simulink model "dual_heater"  (R2023b)
settings: Solver=VariableStepAuto  StartTime=0.0  StopTime=600  FixedStep=1  RelTol=1e-3
values from neighbouring files (symbols this model uses):
  A = 7e-4    (= 0.0007)    [dual_heater1.m]    (also in one_heater1.m = 0.0012)
  alfa = 0.01    [dual_heater1.m]    (also in one_heater1.m = 0.5)
  alfa2 = 0.0075    [dual_heater1.m]
  As = 5e-4    (= 0.0005)    [dual_heater1.m]
  C2K = 273.15    [dual_heater1.m]    (also in one_heater1.m)
  cp = 500    [dual_heater1.m]    (also in one_heater1.m)
  m = 4e-3    (= 0.004)    [dual_heater1.m]    (also in one_heater1.m)
  sig = 5.67e-8    (= 5.67e-08)    [dual_heater1.m]    (also in one_heater1.m)
  T = T + C2K    (= 296.15)    [dual_heater1.m]    (also in one_heater1.m)
  t0 = t0 + C2K    (= 296.15)    [dual_heater1.m]    (also in one_heater1.m)
  U = 10    [dual_heater1.m]    (also in one_heater1.m)
undefined symbols (not defined in the file or in its folder): pow
settings Model: Creator=ondre  LastModifiedBy=ondre

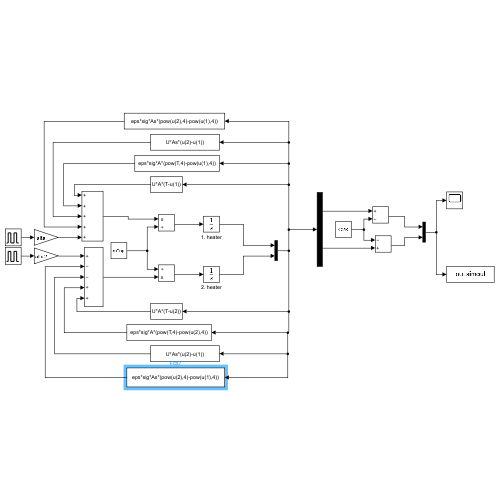
[thumbnail: Simulink's stored preview of the top-level diagram]
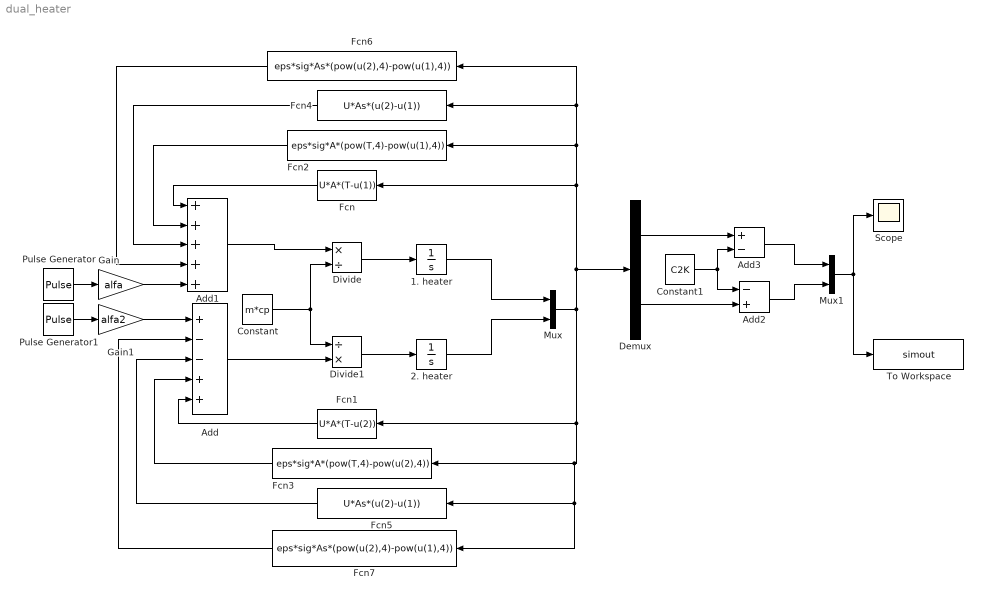
== system dual_heater ==
  1. heater : Integrator  InitialCondition=t0
  2. heater : Integrator  InitialCondition=t0
  Add : Sum  Inputs=+--++
  Add1 : Sum  Inputs=+++++
  Add2 : Sum  Inputs=-+
  Add3 : Sum  Inputs=+-
  Constant : Constant  Value=m*cp
  Constant1 : Constant  Value=C2K
  Demux : Demux  Outputs=2
  Divide : Product  Inputs=*/
  Divide1 : Product  Inputs=/*
  Fcn : Fcn  Expr=U*A*(T-u(1))
  Fcn1 : Fcn  Expr=U*A*(T-u(2))
  Fcn2 : Fcn  Expr=eps*sig*A*(pow(T,4)-pow(u(1),4))
  Fcn3 : Fcn  Expr=eps*sig*A*(pow(T,4)-pow(u(2),4))
  Fcn4 : Fcn  Expr=U*As*(u(2)-u(1))
  Fcn5 : Fcn  Expr=U*As*(u(2)-u(1))
  Fcn6 : Fcn  Expr=eps*sig*As*(pow(u(2),4)-pow(u(1),4))
  Fcn7 : Fcn  Expr=eps*sig*As*(pow(u(2),4)-pow(u(1),4))
  Gain : Gain  Gain=alfa
  Gain1 : Gain  Gain=alfa2
  Mux : Mux  Inputs=2
  Mux1 : Mux  Inputs=2
  Pulse Generator : DiscretePulseGenerator  PulseType=Time based  Period=600  PulseWidth=99
  Pulse Generator1 : DiscretePulseGenerator  PulseType=Time based  Period=600  PulseWidth=99  PhaseDelay=300
  Scope : Scope
  To Workspace : ToWorkspace  VariableName=simout  SaveFormat=Structure With Time  SampleTime=-1
  wires:
  Divide1/1 -> 2. heater/1
  Divide/1 -> 1. heater/1
  Constant/1 -> Divide1/1, Divide/2
  Add1/1 -> Divide/1
  Add/1 -> Divide1/2
  Gain/1 -> Add1/5
  Gain1/1 -> Add/1
  Pulse Generator/1 -> Gain/1
  Pulse Generator1/1 -> Gain1/1
  2. heater/1 -> Mux/2
  1. heater/1 -> Mux/1
  Mux/1 -> Fcn2/1, Fcn6/1, Fcn4/1, Fcn/1, Demux/1, Fcn7/1, Fcn5/1, Fcn3/1, Fcn1/1
  Fcn/1 -> Add1/1
  Fcn1/1 -> Add/5
  Fcn2/1 -> Add1/2
  Fcn3/1 -> Add/4
  Fcn5/1 -> Add/3
  Fcn4/1 -> Add1/3
  Fcn6/1 -> Add1/4
  Fcn7/1 -> Add/2
  Demux/2 -> Add2/2
  Demux/1 -> Add3/1
  Constant1/1 -> Add2/1, Add3/2
  Add3/1 -> Mux1/1
  Add2/1 -> Mux1/2
  Mux1/1 -> Scope/1, To Workspace/1
